simulink model "Z_3Dctrl"  (R2023a)
settings: Solver=ode1  StartTime=0.0  StopTime=inf  FixedStep=0.001  RelTol=1e-3  EnableMultiTasking=on
PostLoadFcn:
  | , if any(exist('dsrtsu_mdlpostloadfcn', 'file') ~= 0), dsrtsu_mdlpostloadfcn('Execute', bdroot); end,
InitFcn:
  | , if any(exist('rtifpga_mdlclblib', 'file') ~= 0), rtifpga_mdlclblib('Init', bdroot); end,
  | [b,a] = butter(6,0.6)
  | z0_default = 0.080001
  | fatness_default = 1
  | offset_default = 0
  | scale_default = 0
  | tic
model workspace (MAT data in the model file):
  Iters = 5
  N_coils = 6
  fatness_default = 1
  running = 0
  z0_default = 0.080001
undefined symbols (not defined in the file or in its folder): a, b, DiscIntNeverNeededParam
libraries: dspstat3 x7, simulink x5, commfilt2 x3, rti2004lib x3, rtilibm x1
(part 3 of 3)

== matlab function Z_3Dctrl/get_plant_input/Z_1dctrl/Wrench scheduling/wrench_scheduler ==
  data: X_SAR input; Y_SAR input; Z_SAR input; PID_XYZ input; PID_out output; wrench_base input; wrench_chunk01 input; wrench_chunk02 input; box_base input; box_chunk01 input; box_chunk02 input; basic_mode input
function PID_out = fcn(X_SAR,Y_SAR,Z_SAR,PID_XYZ,wrench_base,wrench_chunk01,wrench_chunk02,box_base,box_chunk01,box_chunk02,basic_mode)
% Smoothly chooses the wrench matrix to use based on how far away the
% magnet is from the "BASE" wrench's bounding box (on which it was
% trained).
% (08-23-24) For the time being, high Y values mean using Chunk01's wrench,
% and low Y values mean using Chunk02's wrench.

% Read recorded PID gains
x = X_SAR(1);
y = Y_SAR(1);
z = Z_SAR(1);

% Ps = PIDDz_save(:,1);
% Is = PIDDz_save(:,2);
% Douts = PIDDz_save(:,3);
% Dins = PIDDz_save(:,4);
% Zs = PIDDz_save(:,5);
% [~,lowest_index] = min(Zs);
% [~,highest_index] = max(Zs);

% Box range
box_base_xmin = box_base(1,1);
box_base_xmax = box_base(1,1);
box_base_ymin = box_base(1,2);
box_base_ymax = box_base(1,2);

% Chunk01 range
box_chunk01_xmin = box_chunk01(1,1);
box_chunk01_xmax = box_chunk01(1,1);
box_chunk01_ymin = box_chunk01(1,2);
box_chunk01_ymax = box_chunk01(1,2);
box_chunk01_ymean = (box_chunk01_ymin+box_chunk01_ymax)/2;
% Chunk02 range
box_chunk02_xmin = box_chunk02(1,1);
box_chunk02_xmax = box_chunk02(1,1);
box_chunk02_ymin = box_chunk02(1,2);
box_chunk02_ymax = box_chunk02(1,2);
box_chunk02_ymean = (box_chunk02_ymin+box_chunk02_ymax)/2;


% Interpolate if necessary!
if (y <= box_base_ymax && y >= box_base_ymin) || basic_mode==1
    % disp("Inside base chunk!")
    wrench = wrench_base;
elseif basic_mode==2
    xiaodong_wrench =  [0.2500    0.0833    0.1667
                             0    0.1667    0.1667
                       -0.2500    0.0833    0.1667
                       -0.2500   -0.0833    0.1667
                             0   -0.1667    0.1667
                        0.2500   -0.0833    0.1667];
    xiaodong_wrench_XY_scaler = [2.6    0   0
                                   0  2.6   0
                                   0    0   1];
    wrench = xiaodong_wrench * xiaodong_wrench_XY_scaler;

elseif y >= box_base_ymax
    % disp("Start using chunk01!")
    wrench_scale = (y - box_base_ymax)/(box_chunk01_ymean-box_base_ymax);
    wrench = wrench_base*(1-wrench_scale) + wrench_chunk01*(wrench_scale);
else
    % disp("Start using chunk02!")
    wrench_scale = (box_base_ymin - y)/(box_base_ymin - box_chunk02_ymean);
    wrench = wrench_base*(1-wrench_scale) + wrench_chunk02*(wrench_scale);
end

% Apply scaled wrench!
PID_out = wrench*PID_XYZ;

== matlab function Z_3Dctrl/get_plant_input/Z_1dctrl/PID-Vertical/max(0,|dz|-threshold) ==
  data: u_threshold_mm input; u_m input; y output
function y = dz_past_threshold(u_threshold_mm, u_m)
% Input "u" is in metres.
% Input "u_threshold" is in mm.
u_mm = u_m * 1000;    
y = max(0,abs(u_mm) - u_threshold_mm);

== matlab function Z_3Dctrl/get_plant_input/Z_1dctrl/PID-Vertical/PID Gain scheduler/PID selector ==
  data: Zd input; dz input; PIDDz_save input; dz_inner_threshold input; dz_outer_threshold input; PID_out output; P_override input; I_override input; D_override input
function PID_out = fcn(Zd,dz,PIDDz_save,dz_inner_threshold, dz_outer_threshold, P_override,I_override,D_override)
% Interpolates for PID gains based on target Zd, using PID gains that were
% manually tuned at various target heights (with D gain being split into
% "near target height" and "far from target height" values, to allow for
% strong D contribution without risking destabilization near convergence).
% The "D" gain is then chosen between these aforementioned values based on
% how near/far the magnet is to Zd.
%
% Finally, overri

% Read recorded PID gains
Zq = Zd;

Ps = PIDDz_save(:,1);
Is = PIDDz_save(:,2);
Douts = PIDDz_save(:,3);
Dins = PIDDz_save(:,4);
Zs = PIDDz_save(:,5);
[~,lowest_index] = min(Zs);
[~,highest_index] = max(Zs);


% Interpolate if necessary!
if Zd <= Zs(lowest_index)
    % disp("Below 2mm!")
    P_final = Ps(lowest_index);
    I_final = Is(lowest_index);
    Dout_final = Douts(lowest_index);
    Din_final  = Dins(lowest_index);
elseif Zd >= Zs(highest_index)
    % disp("Above 5mm!")
    P_final = Ps(highest_index);
    I_final = Is(highest_index);
    Dout_final = Douts(highest_index);
    Din_final  = Dins(highest_index);
else
    % disp("Interpolate!")
    P_final     = interp1(Zs,Ps,Zq,'spline');
    I_final     = interp1(Zs,Is,Zq,'spline');
    Dout_final  = interp1(Zs,Douts,Zq,'spline');
    Din_final   = interp1(Zs,Dins,Zq,'spline');
end



% Choose between "inner" and "outer" D gains
dz_mm = dz * 1000;

if abs(dz_mm) <= dz_inner_threshold
    % disp("Within inner threshold")
    D_final = Din_final;
elseif abs(dz_mm) >= dz_outer_threshold
    % disp("Beyond outer threshold")
    D_final = Dout_final;
else
    % disp("In between; interpolate!")
    D_final = ( Dout_final- Din_final)*(abs(dz_mm) - dz_inner_threshold)/(dz_outer_threshold - dz_inner_threshold) +  Din_final;
end


% Apply overrides (if any)
if ~isnan(P_override)
    P_final = P_override;
end
if ~isnan(I_override)
    I_final = I_override;
end
if ~isnan(D_override)
    D_final = D_override;
end
PID_out = [P_final, I_final, D_final];
